simulink model "Apollo_LM"  (R2018b)
settings: Solver=VariableStepAuto  StartTime=0.0  StopTime=100  RelTol=1e-3
model workspace (MATLAB code in the model file):
  | g_M = 1.62; %m/s gravity at moon surface
  | J = 1e5; %kg*m*m
values from neighbouring files (symbols this model uses):
  Gamma = h*k1*[1;h/2; k2*h^2/6]    [Apollo_LM_design.m]    (also in Apollo_LM_design_observer.m; Apollo_LM_share.m)
  h = 1    [Apollo_LM_design.m]    (also in Apollo_LM_design_observer.m; Apollo_LM_share.m = 0.25; L11.m = 0.1; cart-oscillator-input-design.m = 0.5)
  L = L_a    [Apollo_LM_design.m]    (also in Apollo_LM_design_observer.m; Apollo_LM_share.m; gantry_crane_equations_of_motion.m = Tt+Tc - V)
  l0 = 1/(C*inv((eye(3)-Phic))*Gamma)    [Apollo_LM_design.m]    (also in Apollo_LM_design_observer.m; Apollo_LM_share.m)
  Phi = [1, 0 , 0 ... (first row only)    [Apollo_LM_design.m]    (also in Apollo_LM_design_observer.m; Apollo_LM_share.m)
  Phic = Phi - Gamma*L    [Apollo_LM_design.m]    (also in Apollo_LM_design_observer.m; Apollo_LM_share.m)
settings Model: Creator=kjartan  LastModifiedBy=kjartan

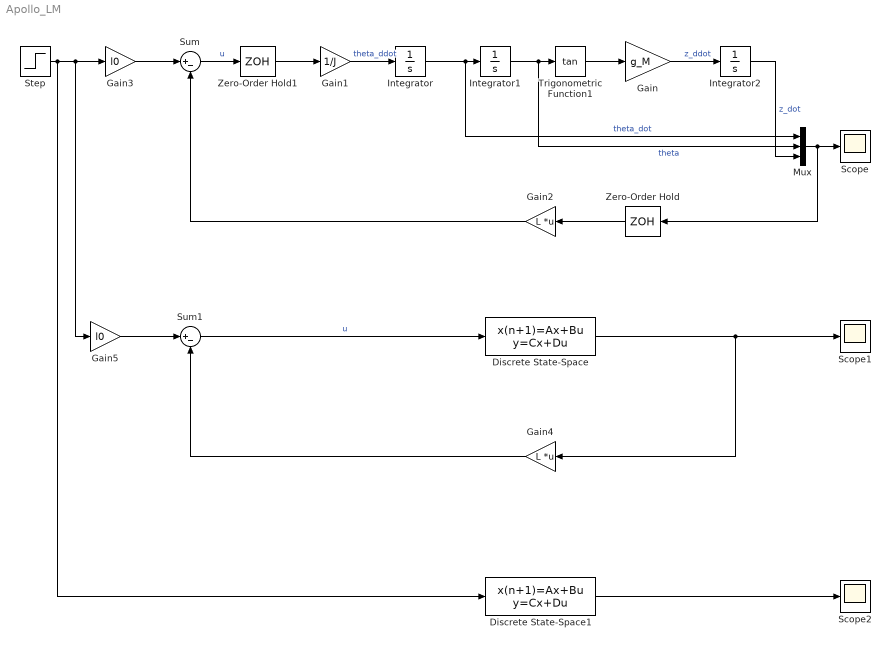
== system Apollo_LM ==
  Discrete State-Space : DiscreteStateSpace  A=Phi  B=Gamma  C=eye(3)  D=zeros(3,1)  SampleTime=h
  Discrete State-Space1 : DiscreteStateSpace  A=Phic  B=Gamma*l0  C=eye(3)  D=zeros(3,1)  SampleTime=h
  Gain : Gain  Gain=g_M
  Gain1 : Gain  Gain=1/J
  Gain2 : Gain  Gain=L  Multiplication=Matrix(K*u)
  Gain3 : Gain  Gain=l0
  Gain4 : Gain  Gain=L  Multiplication=Matrix(K*u)
  Gain5 : Gain  Gain=l0
  Integrator : Integrator
  Integrator1 : Integrator
  Integrator2 : Integrator
  Mux : Mux  Inputs=3
  Scope : Scope
  Scope1 : Scope
  Scope2 : Scope
  Step : Step  SampleTime=0
  Sum : Sum  Inputs=|+-
  Sum1 : Sum  Inputs=|+-
  Trigonometric Function1 : Trigonometry  Operator=tan
  Zero-Order Hold : ZeroOrderHold  SampleTime=h
  Zero-Order Hold1 : ZeroOrderHold  SampleTime=h
  wires:
  Integrator1/1 -> Mux/2, Trigonometric Function1/1  "theta"
  Trigonometric Function1/1 -> Gain/1
  Integrator/1 -> Mux/1, Integrator1/1  "theta_dot"
  Gain1/1 -> Integrator/1  "theta_ddot"
  Gain/1 -> Integrator2/1  "z_ddot"
  Mux/1 -> Zero-Order Hold/1, Scope/1
  Integrator2/1 -> Mux/3  "z_dot"
  Sum/1 -> Zero-Order Hold1/1  "u"
  Zero-Order Hold/1 -> Gain2/1
  Gain2/1 -> Sum/2
  Gain3/1 -> Sum/1
  Zero-Order Hold1/1 -> Gain1/1
  Discrete State-Space/1 -> Gain4/1, Scope1/1
  Step/1 -> Discrete State-Space1/1, Gain5/1, Gain3/1
  Gain5/1 -> Sum1/1
  Gain4/1 -> Sum1/2
  Sum1/1 -> Discrete State-Space/1  "u"
  Discrete State-Space1/1 -> Scope2/1
